simulink model "BatteryModuleModelDifferentialEquationsForMPC"  (R2023b)
settings: Solver=VariableStepAuto  StartTime=0.0  StopTime=33749  RelTol=1e-3
values from neighbouring files (symbols this model uses):
  C1 = 12.6138    [DPBatteryDynamics.m]    (also in DPBatteryModuleDynamics.m = 174.354594213; MPCControllerForModuleSim.m = 174.354594213; StateSpaceScript.m; TubeBasedMPCControllerForModuleSim.m = 174.354594213)
  Cc = 62.7    [DPBatteryDynamics.m]    (also in DPBatteryModuleDynamics.m = 2059.88437317; MPCControllerForModuleSim.m = 2059.88437317; StateSpaceScript.m; TubeBasedMPCControllerForModuleSim.m = 2059.88437317)
  Cn = 78    [DPBatteryDynamics.m]    (also in DPBatteryModuleDynamics.m = 156; MPCControllerForModuleSim.m = 156; StateSpaceScript.m; TubeBasedMPCControllerForModuleSim.m = 156)
  Cs = 4.5    [DPBatteryDynamics.m]    (also in DPBatteryModuleDynamics.m = 31.8813725212; MPCControllerForModuleSim.m = 31.8813725212; StateSpaceScript.m; TubeBasedMPCControllerForModuleSim.m = 31.8813725212)
  ENom = 992623.375585428    (= 992623.375585)    [DPBatteryDynamics.m]    (also in DPBatteryModuleDynamics.m = 24521235.1894; FMINCONControllerForCellSim.m; MPCControllerForModuleSim.m = 24521235.1894; TubeBasedMPCControllerForCellSim.m)
  IBar = sqrt(Cc*(TcBar - TsBar) / (Rc*Cc*(R1+R0)))    [StateSpaceScript.m]
  R0 = 0.0099131    [DPBatteryDynamics.m]    (also in DPBatteryModuleDynamics.m = 0.000127631043389; FMINCONControllerForCellSim.m = 0.00292724690916; MPCControllerForModuleSim.m = 0.000127631043389; StateSpaceScript.m)
  R1 = 3e-4    (= 0.0003)    [DPBatteryDynamics.m]    (also in DPBatteryModuleDynamics.m = 0.00360795873337; MPCControllerForModuleSim.m = 0.00360795873337; StateSpaceScript.m; TubeBasedMPCControllerForModuleSim.m = 0.00360795873337)
  Rc = 1.94    [DPBatteryDynamics.m]    (also in DPBatteryModuleDynamics.m = 14.480191951; MPCControllerForModuleSim.m = 14.480191951; StateSpaceScript.m; TubeBasedMPCControllerForModuleSim.m = 14.480191951)
  Ru = 15    [DPBatteryDynamics.m]    (also in DPBatteryModuleDynamics.m = 8.86466905699; MPCControllerForModuleSim.m = 8.86466905699; StateSpaceScript.m; TubeBasedMPCControllerForModuleSim.m = 8.86466905699)
  Tf = 20    [DPBatteryDynamics.m]    (also in DPBatteryModuleDynamics.m; MPCControllerForModuleSim.m; RHC_test.m; StateSpaceScript.m)
  TsBar = (Ru*TcBar + Rc*Tf) / (Ru+Rc)    (= 37.7095631641)    [StateSpaceScript.m]
  x0 = [1; 0; Tf; Tf]    [RHC_test.m]    (also in RunModuleDP.m = [1 0 20 20 1]'; StateSpaceScript.m = [1 0 Tf Tf]')
undefined symbols (not defined in the file or in its folder): Discrete, exportVar, linsys34, MPCControllerForModuleSim, Time
libraries: simulink x3, ctrlSharedLib x1
settings Model: Creator=adamb  LastModifiedBy=Adam
settings DataIOCC: ExternalInput=tp212d7339_d485_4be7_bfbc_c7c176cfddaf(1)  OutputTimes=SDO_OutputTimes  ReturnWorkspaceOutputsName=SDOSimTest_Log

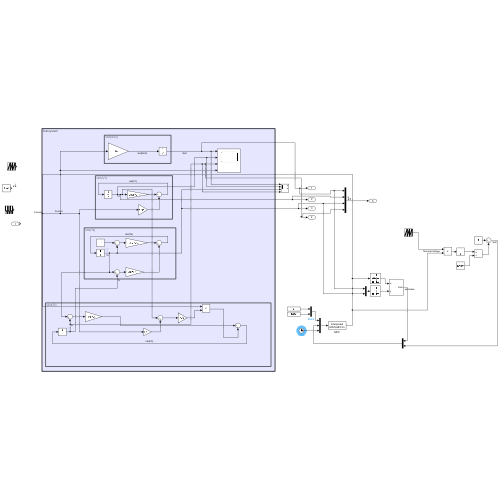
[thumbnail: Simulink's stored preview of the top-level diagram]
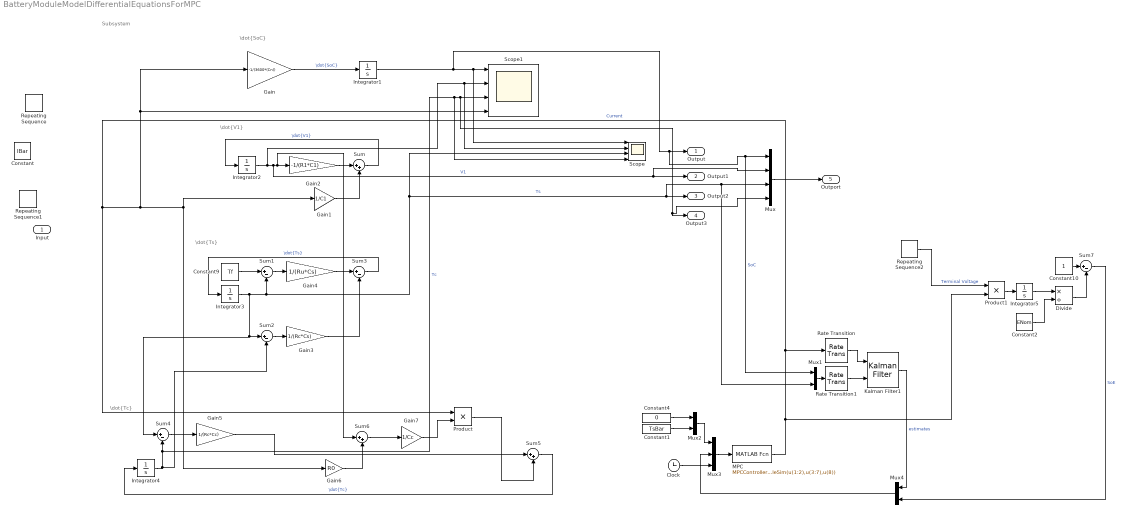
== system BatteryModuleModelDifferentialEquationsForMPC ==
  note: Subsystem
  note: \dot{V1}
  note: \dot{SoC}
  note: \dot{Ts}
  note: \dot{Tc}
  Input : Inport
  Clock : Clock
  Constant : Constant  Value=IBar
  Constant1 : Constant  Value=TsBar
  Constant10 : Constant
  Constant2 : Constant  Value=ENom
  Constant4 : Constant  Value=0
  Constant9 : Constant  Value=Tf
  Divide : Product  Inputs=*/
  Gain : Gain  Gain=-1/(3600*(Cn))
  Gain1 : Gain  Gain=1/C1
  Gain2 : Gain  Gain=-1/(R1*C1)
  Gain3 : Gain  Gain=1/(Rc*Cs)
  Gain4 : Gain  Gain=1/(Ru*Cs)
  Gain5 : Gain  Gain=1/(Rc*Cc)
  Gain6 : Gain  Gain=R0
  Gain7 : Gain  Gain=1/Cc
  Integrator1 : Integrator  InitialCondition=1
  Integrator2 : Integrator
  Integrator3 : Integrator  InitialCondition=Tf
  Integrator4 : Integrator  InitialCondition=Tf
  Integrator5 : Integrator
  Kalman Filter1 : ctrlSharedLib/Kalman Filter  TimeDomain=Discrete-Time  UseCurrentEstimator=on  ModelSource=Individual A, B, C, D matrices  ModelSourceVariable=ss(0.95,1,1,0,1)  A=linsys34.A  B=linsys34.B  C=[1 0 0 0;0 0 1 0]  D=zeros(2,1)  NumberOfStates=1  NumberOfInputs=1  NumberOfOutputs=1  InitialEstimateSource=Dialog  X0=x0(1:4)  P0=10  UseK=off  UseGH=off  NumberOfProcessNoiseInputs=1  G=1  TimeInvariantG=on  H=0  TimeInvariantH=on  Q=10  TimeInvariantQ=on  R=0.3  TimeInvariantR=on  N=0  TimeInvariantN=on  AddInputPort=on  AddEnablePort=off  OutputEstimatedY=off  OutputP=off  Ts=1
  MPC : MATLABFcn  MATLABFcn=MPCControllerForModuleSim(u(1:2),u(3:7),u(8))
  Mux : Mux
  Mux1 : Mux  Inputs=2
  Mux2 : Mux  Inputs=2
  Mux3 : Mux  Inputs=3
  Mux4 : Mux  Inputs=2
  Product : Product
  Product1 : Product
  Rate Transition : RateTransition  OutPortSampleTime=1
  Rate Transition1 : RateTransition  OutPortSampleTime=1
  Repeating Sequence : simulink/Sources/Repeating Sequence  rep_seq_t=1:4e4  rep_seq_y=[DPModuleSolution DPModuleSolution(end-9999:end) DPModuleSolution(end-9999:end)]
  Repeating Sequence1 : simulink/Sources/Repeating Sequence  rep_seq_t=[0 5500 5501 30696 30697 45097]  rep_seq_y=[40 40 IBar IBar 0 0]
  Repeating Sequence2 : simulink/Sources/Repeating Sequence  rep_seq_t=exportVar{1}.Values.Time'  rep_seq_y=exportVar{1}.Values.Data(:,1)'
  Scope : Scope  NumInputPorts=4
  Scope1 : Scope  NumInputPorts=4
  Sum : Sum  Inputs=|++
  Sum{1..4,7} (5 alike) : Sum  Inputs=|+-
  Sum5 : Sum  Inputs=|++
  Sum6 : Sum  Inputs=|++
  Output : Outport
  Output1 : Outport  Port=2
  Output2 : Outport  Port=3
  Output3 : Outport  Port=4
  Outport : Outport  Port=5
  wires:
  Sum3/1 -> Integrator3/1  "\\dot{Ts}"
  Sum2/1 -> Gain3/1
  Sum1/1 -> Gain4/1
  Product/1 -> Sum5/2
  Gain/1 -> Integrator1/1  "\\dot{SoC}"
  Gain2/1 -> Sum/1
  Gain7/1 -> Product/2
  Gain5/1 -> Sum5/1
  Constant9/1 -> Sum1/1
  Integrator2/1 -> Mux/2, Output1/1, Sum6/1, Gain2/1, Scope/2, Scope1/2  "V1"
  Gain6/1 -> Sum6/2
  Gain3/1 -> Sum3/2
  Sum4/1 -> Gain5/1
  Integrator3/1 -> Sum4/1, Sum2/1, Mux1/2, Mux/3, Output2/1, Scope/3, Sum1/2  "Ts"
  Sum5/1 -> Integrator4/1  "\\dot{Tc}"
  Integrator1/1 -> Mux1/1, Mux/1, Output/1, Scope/1, Scope1/1  "SoC"
  Integrator4/1 -> Sum2/2, Scope/4, Mux/4, Output3/1, Scope1/3, Sum4/2  "Tc"
  Sum/1 -> Integrator2/1  "\\dot{V1}"
  Sum6/1 -> Gain7/1
  Gain4/1 -> Sum3/1
  Gain1/1 -> Sum/2
  Mux/1 -> Outport/1
  MPC/1 -> Product1/2, Rate Transition/1, Product/1, Gain1/1, Gain6/1, Scope1/4, Gain/1  "Current"
  Mux1/1 -> Rate Transition1/1
  Rate Transition/1 -> Kalman Filter1/1
  Rate Transition1/1 -> Kalman Filter1/2
  Mux2/1 -> Mux3/1
  Constant4/1 -> Mux2/1
  Constant1/1 -> Mux2/2
  Clock/1 -> Mux3/3
  Mux4/1 -> Mux3/2
  Kalman Filter1/1 -> Mux4/1  "estimates"
  Divide/1 -> Sum7/2
  Integrator5/1 -> Divide/1
  Product1/1 -> Integrator5/1
  Constant2/1 -> Divide/2
  Constant10/1 -> Sum7/1
  Repeating Sequence2/1 -> Product1/1  "Terminal Voltage"
  Sum7/1 -> Mux4/2  "SoE"
  Mux3/1 -> MPC/1
